simulink model "Morten_dq_control"  (R2015b)
settings: Solver=VariableStepAuto  StartTime=0.0  StopTime=10.0  RelTol=1e-3
libraries: powerlib_meascontrol x2
settings Model: Creator=Morten  LastModifiedBy=Morten

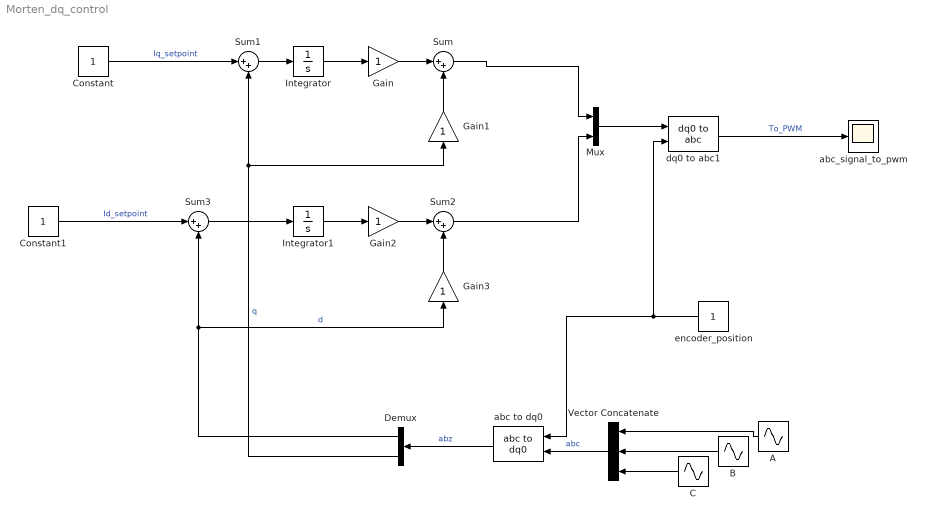
== system Morten_dq_control ==
  A : Sin  SampleTime=0
  B : Sin  Phase=-2/3*pi  SampleTime=0
  C : Sin  Phase=2/3*pi  SampleTime=0
  Constant : Constant
  Constant1 : Constant
  Demux : Demux  Outputs=2
  Gain{,1..3} (4 alike) : Gain
  Integrator : Integrator
  Integrator1 : Integrator
  Mux : Mux  Inputs=2
  Sum{,1..3} (4 alike) : Sum  Inputs=|++
  Vector Concatenate : Concatenate  NumInputs=3
  abc to dq0 : powerlib_meascontrol/Transformations/abc to dq0  Alignment=90 degrees behind phase A axis
  abc_signal_to_pwm : Scope
  dq0 to abc1 : powerlib_meascontrol/Transformations/dq0 to abc  Alignment=90 degrees behind phase A axis
  encoder_position : Constant
  wires:
  Integrator/1 -> Gain/1
  Gain1/1 -> Sum/2
  Gain/1 -> Sum/1
  Sum1/1 -> Integrator/1
  Constant/1 -> Sum1/1  "Iq_setpoint"
  B/1 -> Vector Concatenate/2
  C/1 -> Vector Concatenate/3
  A/1 -> Vector Concatenate/1
  Vector Concatenate/1 -> abc to dq0/1  "abc"
  abc to dq0/1 -> Demux/1  "abz"
  Integrator1/1 -> Gain2/1
  Gain3/1 -> Sum2/2
  Gain2/1 -> Sum2/1
  Sum3/1 -> Integrator1/1
  Constant1/1 -> Sum3/1  "Id_setpoint"
  Sum2/1 -> Mux/2
  Mux/1 -> dq0 to abc1/1
  Sum/1 -> Mux/1
  Demux/1 -> Gain3/1, Sum3/2  "d"
  Demux/2 -> Gain1/1, Sum1/2  "q"
  dq0 to abc1/1 -> abc_signal_to_pwm/1  "To_PWM"
  encoder_position/1 -> dq0 to abc1/2, abc to dq0/2
